simulink model "AutomaticFog_Detector"  (R2024a)
settings: Solver=FixedStepDiscrete  StartTime=0.0  StopTime=10.0  RelTol=1e-3  EnableMultiTasking=on
values from neighbouring files (symbols this model uses):
  Dem_EventStatusType : value not decoded    [dict.sldd]
libraries: autosarlibnvm x2, autosarlibdem x1
settings Model: DataDictionary=dict.sldd  Creator=Administrator  LastModifiedBy=Administrator
settings OptimizationCC: DefaultParameterBehavior=Inlined  EnhancedBackFolding=on  PassReuseOutputArgsAs=Individual arguments  ZeroExternalMemoryAtStartup=off  ZeroInternalMemoryAtStartup=off  OptimizeBlockOrder=speed  DifferentSizesBufferReuse=on  OptimizationCustomize=off  EfficientTunableParamExpr=on
settings DebuggingCC: ParameterTunabilityLossMsg=error
settings SFSimCC: MATLABDynamicMemAlloc=off
settings RTWCC: Description=AUTOSAR  SystemTargetFile=autosar.tlc  GenCodeOnly=on  TemplateMakefile=ert_default_tmf  DataTypeReplacement=CDataTypesFixedWidth
settings CodeAppCC: ForceParamTrailComments=on  IgnoreCustomStorageClasses=off  OperatorAnnotations=on  SimulinkDataObjDesc=on  SFDataObjDesc=on  InsertBlockDesc=on
settings STFCustomTargetCC: MultiwordLength=256  ParMdlRefBuildCompliant=on  CompOptLevelCompliant=on  IncludeMdlTerminateFcn=off  CombineOutputUpdateFcns=on  SuppressErrorStatus=on  ERTCustomFileBanners=on  SupportNonFinite=off  SupportComplex=off  SupportContinuousTime=off  SupportNonInlinedSFcns=off  RemoveResetFunc=on  MATLABClassNameForMDSCustomization=Simulink.SoftwareTarget.ERTCustomization  AutosarCompliant=on  GRTInterface=off  LookupTableObjectStructAxisOrder=2,1,3,4,...  LUTObjectStructOrderEvenSpacing=Size,Table,Breakpoints  SystemTargetFile=autosar.tlc
settings ERTTargetCC: TargetLangStandard=C99 (ISO)  ConcurrentExecutionCompliant=off  IncludeMdlTerminateFcn=off  SuppressErrorStatus=on  SupportNonFinite=off  SupportComplex=off  ModelStepFunctionPrototypeControlCompliant=off  CPPClassGenCompliant=off  AutosarCompliant=on  LookupTableObjectStructAxisOrder=2,1,3,4,...  LUTObjectStructOrderEvenSpacing=Size,Table,Breakpoints  InlinedParameterPlacement=NonHierarchical  ERTCustomFileTemplate=example_file_process.tlc  BooleanTrueId=TRUE  BooleanFalseId=FALSE

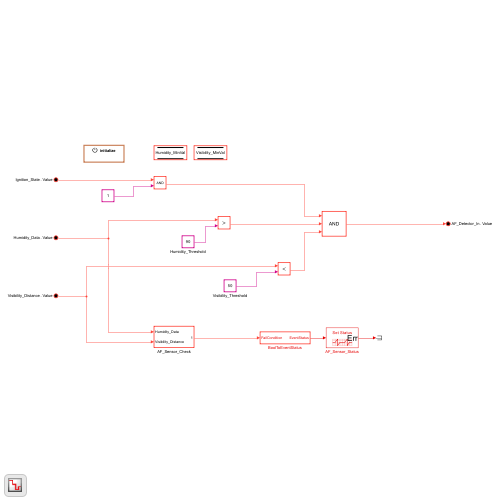
[thumbnail: Simulink's stored preview of the top-level diagram]
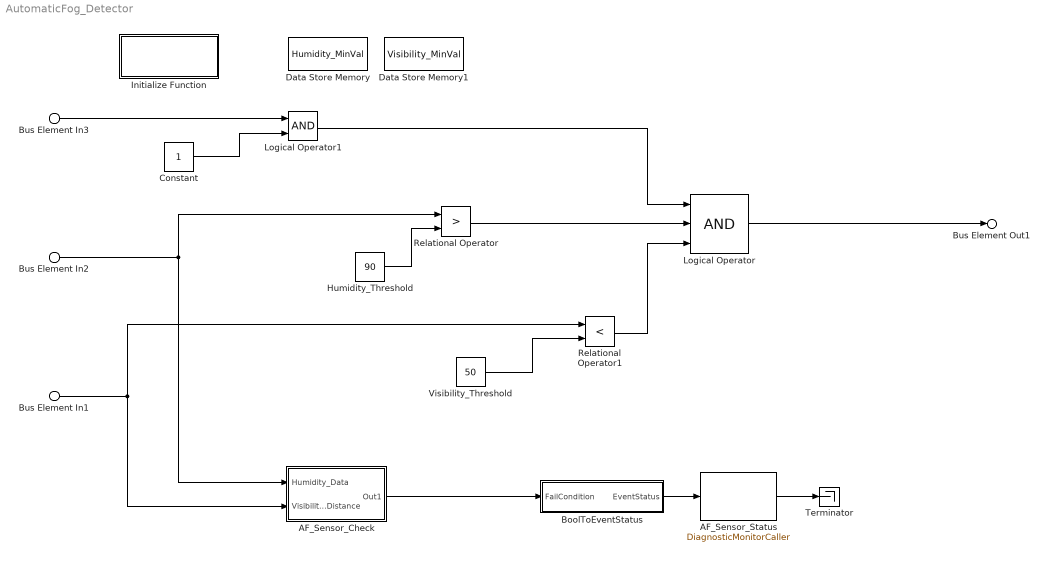
== system AutomaticFog_Detector ==
  Bus Element In3 : Inport  Description=|  PortName=Ignition_State  Element=Value
      | Ignition State:
      | 0: OFF
      | 1: ON
  Bus Element In1 : Inport  Port=2  PortName=Visibility_Distance  Element=Value
  Bus Element In2 : Inport  Port=3  PortName=Humidity_Data  Element=Value
  AF_Sensor_Check : Subsystem
  AF_Sensor_Status : autosarlibdem/DiagnosticMonitorCaller  PortName=AF_Detector  Operation=SetEventStatus  Datatype=Enum: Dem_EventStatusType  st=-1  ServiceImpl=autosar.bsw.DemDiagnosticMonitor  SyncToSchema=off
  BoolToEventStatus : Subsystem
  Constant : Constant
  Data Store Memory : DataStoreMemory  DataStoreName=Humidity_MinVal  WriteAfterWriteMsg=warning  ShowAdditionalParam=off
  Data Store Memory1 : DataStoreMemory  DataStoreName=Visibility_MinVal  WriteAfterWriteMsg=warning  ShowAdditionalParam=off
  Humidity_Threshold : Constant  Value=90
  Initialize Function : Subsystem  TreatAsAtomicUnit=on
  Logical Operator : Logic  Inputs=3  AllPortsSameDT=off  OutDataTypeStr=boolean
  Logical Operator1 : Logic  AllPortsSameDT=off  OutDataTypeStr=boolean
  Relational Operator : RelationalOperator  Operator=>  OutDataTypeStr=boolean  RndMeth=Simplest  InputSameDT=off
  Relational Operator1 : RelationalOperator  Operator=<  OutDataTypeStr=boolean  RndMeth=Simplest  InputSameDT=off
  Terminator : Terminator
  Visibility_Threshold : Constant  Value=50
  Bus Element Out1 : Outport  PortName=AF_Detector_In  Element=Value
  wires:
  Relational Operator1/1 -> Logical Operator/3
  Visibility_Threshold/1 -> Relational Operator1/2
  Bus Element In2/1 -> Relational Operator/1, AF_Sensor_Check/1(Humidity_Data)
  Logical Operator/1 -> Bus Element Out1/1
  Bus Element In1/1 -> AF_Sensor_Check/2(Visibility_Distance), Relational Operator1/1
  AF_Sensor_Check/1(Out1) -> BoolToEventStatus/1(FailCondition)
  Logical Operator1/1 -> Logical Operator/1
  Bus Element In3/1 -> Logical Operator1/1
  Constant/1 -> Logical Operator1/2
  Humidity_Threshold/1 -> Relational Operator/2
  Relational Operator/1 -> Logical Operator/2
  BoolToEventStatus/1(EventStatus) -> AF_Sensor_Status/1
  AF_Sensor_Status/1 -> Terminator/1

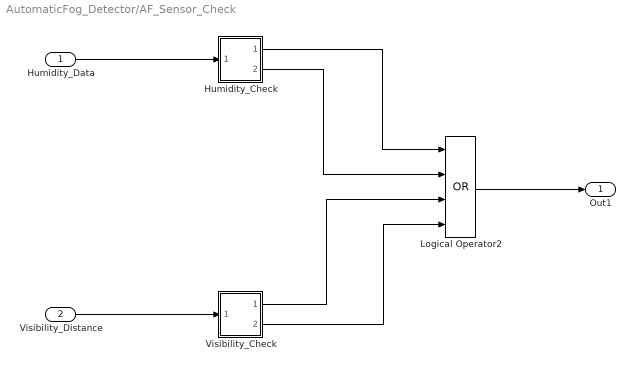
== system AutomaticFog_Detector/AF_Sensor_Check ==
  Humidity_Data : Inport
  Visibility_Distance : Inport  Port=2
  Humidity_Check : Subsystem
  Logical Operator2 : Logic  Operator=OR  Inputs=4  AllPortsSameDT=off  OutDataTypeStr=boolean
  Visibility_Check : Subsystem
  Out1 : Outport
  wires:
  Logical Operator2/1 -> Out1/1
  Visibility_Check/1(Out1) -> Logical Operator2/3
  Visibility_Check/2(Out2) -> Logical Operator2/4
  Humidity_Data/1 -> Humidity_Check/1(In1)
  Humidity_Check/2(Out2) -> Logical Operator2/2
  Humidity_Check/1(Out1) -> Logical Operator2/1
  Visibility_Distance/1 -> Visibility_Check/1(In1)

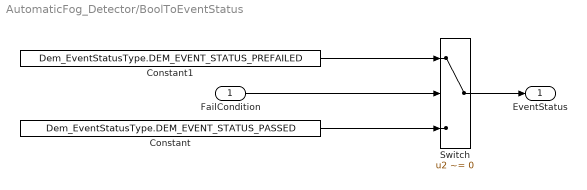
== system AutomaticFog_Detector/BoolToEventStatus ==
  FailCondition : Inport
  Constant : Constant  Value=Dem_EventStatusType.DEM_EVENT_STATUS_PASSED
  Constant1 : Constant  Value=Dem_EventStatusType.DEM_EVENT_STATUS_PREFAILED
  Switch : Switch  Criteria=u2 ~= 0  SaturateOnIntegerOverflow=off  InputSameDT=off
  EventStatus : Outport  VectorParamsAs1DForOutWhenUnconnected=off
  wires:
  FailCondition/1 -> Switch/2
  Constant/1 -> Switch/3
  Constant1/1 -> Switch/1
  Switch/1 -> EventStatus/1

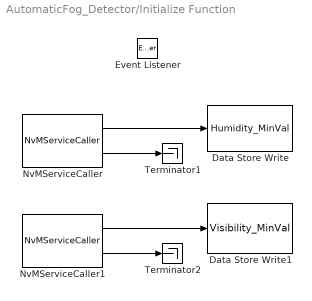
== system AutomaticFog_Detector/Initialize Function ==
  Data Store Write : DataStoreWrite  DataStoreName=Humidity_MinVal  IndexOptions=Index vector (dialog)  Indices=1  OutputSizes=1
  Data Store Write1 : DataStoreWrite  DataStoreName=Visibility_MinVal  IndexOptions=Index vector (dialog)  Indices=1  OutputSizes=1
  Event Listener : EventListener  DisableCoverage=on  EventName=reset
  NvMServiceCaller : autosarlibnvm/NvMServiceCaller  PortName=Humidity_MinVal  Operation=ReadBlock  ArgumentSpecification=uint8(0)  st=-1  ServiceImpl=autosar.bsw.NvMService  SyncToSchema=off
  NvMServiceCaller1 : autosarlibnvm/NvMServiceCaller  PortName=Visibility_MinVal  Operation=ReadBlock  ArgumentSpecification=uint8(0)  st=-1  ServiceImpl=autosar.bsw.NvMService  SyncToSchema=off
  Terminator1 : Terminator
  Terminator2 : Terminator
  wires:
  NvMServiceCaller/1 -> Data Store Write/1
  NvMServiceCaller/2 -> Terminator1/1
  NvMServiceCaller1/2 -> Terminator2/1
  NvMServiceCaller1/1 -> Data Store Write1/1

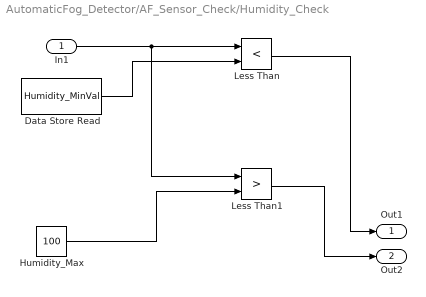
== system AutomaticFog_Detector/AF_Sensor_Check/Humidity_Check ==
  In1 : Inport
  Data Store Read : DataStoreRead  DataStoreName=Humidity_MinVal  IndexOptions=Index vector (dialog)  Indices=1  OutputSizes=1
  Humidity_Max : Constant  Value=100
  Less Than : RelationalOperator  Operator=<  OutDataTypeStr=boolean  RndMeth=Simplest  InputSameDT=off
  Less Than1 : RelationalOperator  Operator=>  OutDataTypeStr=boolean  RndMeth=Simplest  InputSameDT=off
  Out1 : Outport
  Out2 : Outport  Port=2
  wires:
  Data Store Read/1 -> Less Than/2
  Less Than/1 -> Out1/1
  Humidity_Max/1 -> Less Than1/2
  In1/1 -> Less Than1/1, Less Than/1
  Less Than1/1 -> Out2/1

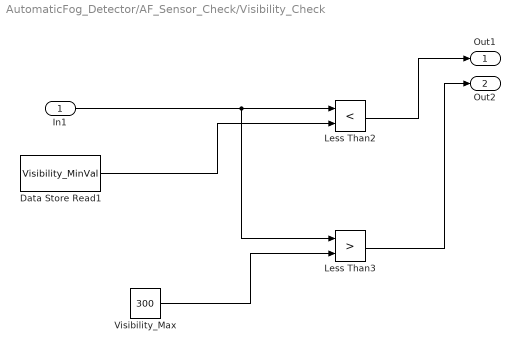
== system AutomaticFog_Detector/AF_Sensor_Check/Visibility_Check ==
  In1 : Inport
  Data Store Read1 : DataStoreRead  DataStoreName=Visibility_MinVal  IndexOptions=Index vector (dialog)  Indices=1  OutputSizes=1
  Less Than2 : RelationalOperator  Operator=<  OutDataTypeStr=boolean  RndMeth=Simplest  InputSameDT=off
  Less Than3 : RelationalOperator  Operator=>  OutDataTypeStr=boolean  RndMeth=Simplest  InputSameDT=off
  Visibility_Max : Constant  Value=300
  Out1 : Outport
  Out2 : Outport  Port=2
  wires:
  Less Than3/1 -> Out2/1
  Data Store Read1/1 -> Less Than2/2
  Visibility_Max/1 -> Less Than3/2
  In1/1 -> Less Than3/1, Less Than2/1
  Less Than2/1 -> Out1/1
